simulink model "Dynamixel_Control_Validation_SpeedMode_2023a"  (R2023a)
settings: Solver=ode4  StartTime=0.0  StopTime=10  FixedStep=0.01  RelTol=1e-6  AbsTol=1e-6
undefined symbols (not defined in the file or in its folder): DiscIntNeverNeededParam
libraries: simulink x3, nvidiaSharedBlocks x1
settings Model: PauseTimes=45  Creator=SPOT  LastModifiedBy=SPOT
settings OptimizationCC: EnhancedBackFolding=on  PassReuseOutputArgsAs=Individual arguments  ZeroExternalMemoryAtStartup=off  ZeroInternalMemoryAtStartup=off  MaxStackSize=64  OptimizeBlockOrder=speed  DifferentSizesBufferReuse=on  OptimizationCustomize=off  EfficientTunableParamExpr=on
settings DebuggingCC: ParameterTunabilityLossMsg=error
settings HardwareCC: ProdBitPerLong=64  ProdLargestAtomicInteger=LongLong  ProdLargestAtomicFloat=Double  ProdLongLongMode=on  ProdHWDeviceType=ARM Compatible->ARM 64-bit (LP64)
settings SFSimCC: MATLABDynamicMemAlloc=off
settings RTWCC: Description=Embedded Coder  SystemTargetFile=ert.tlc  HardwareBoard=NVIDIA Jetson  TLCOptions="-aInlineSetEventsForThisBaseRateFcn=TLC_FALSE -aSuppressMultiTaskScheduler=TLC_FALSE  -aRateBasedStepFcn=0"  TemplateMakefile=ert_default_tmf  TargetLang=C++
settings CodeAppCC: ForceParamTrailComments=on  IgnoreCustomStorageClasses=off  OperatorAnnotations=on  SimulinkDataObjDesc=on  SFDataObjDesc=on  InsertBlockDesc=on
settings ERTTargetCC: MatFileLogging=on  SupportContinuousTime=on  SupportVariableSizeSignals=on

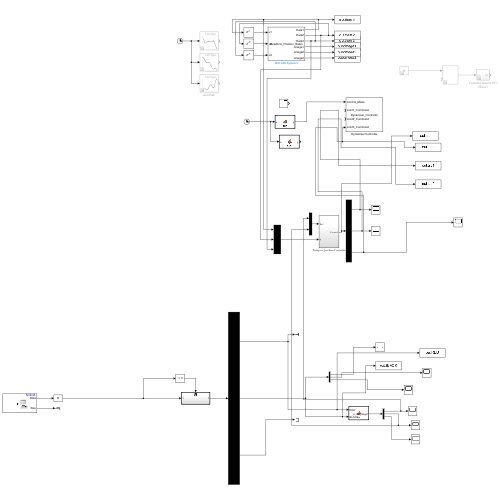
[thumbnail: Simulink's stored preview of the top-level diagram]
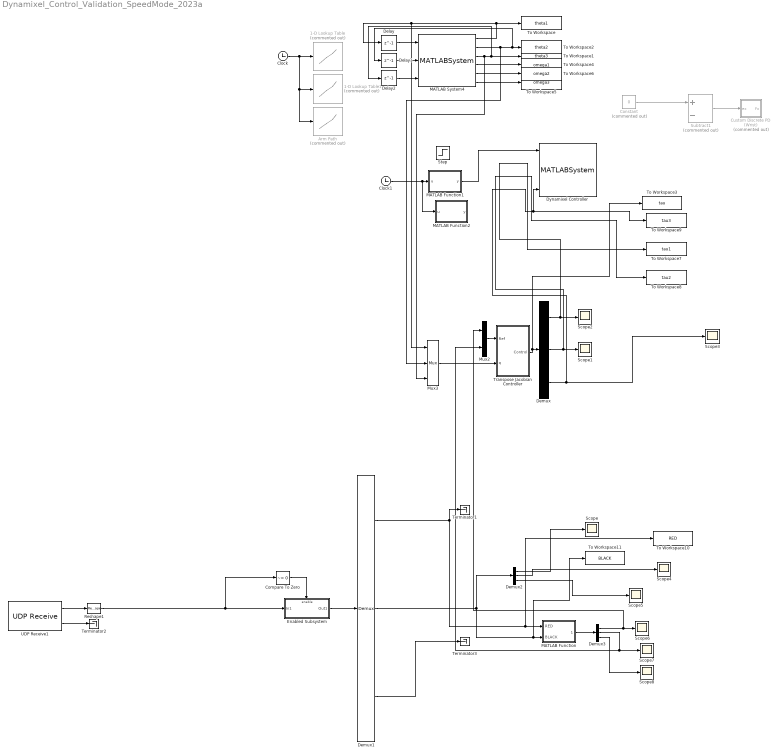
== system Dynamixel_Control_Validation_SpeedMode_2023a ==
  1-D Lookup Table : Lookup_n-D  Commented=on  NumberOfTableDimensions=1  BreakpointsForDimension1=|  Table=|  InternalRulePriority=Speed  RndMeth=Simplest
      BreakpointsForDimension1=|
      | [0
      | 0.300000000000000
      | 0.600000000000000
      | 0.900000000000000
      | 1.20000000000000
      | 1.50000000000000
      | 1.80000000000000
      | 2.10000000000000
      | 2.40000000000000
      | 2.70000000000000
      | 3
      | 3.30000000000000
      | 3.60000000000000
      | 3.90000000000000
      | 4.20000000000000
      | 4.50000000000000
      | 4.80000000000000
      | 5.10000000000000
      | 5.40000000000000
      | 5.70000000000000
      | 6
      | 6.30000000000000
      | 6.60000000000000
      | 6.90000000000000
      | 7.20000000000000
      | 7.50000000000000
      | 7.80000000000000
      | 8.10000000000000
      | 8.40000000000000
      | 8.70000000000000
      | 9
      | 9.30000000000000
      | 9.60000000000000
      | 9.90000000000000
      | 10.2000000000000
      | 10.5000000000000
      | 10.8000000000000
      | 11.1000000000000
      | 11.4000000000000
      | 11.7000000000000
      | 12
      | 12.3000000000000
      | 12.6000000000000
      | 12.9000000000000
      | 13.2000000000000
      | 13.5000000000000
      | 13.8000000000000
      | 14.1000000000000
      | 14.4000000000000
      | 14.7000000000000
      | 15
      | 15.3000000000000
      | 15.6000000000000
      | 15.9000000000000
      | 16.2000000000000
      | 16.5000000000000
      | 16.8000000000000
      | 17.1000000000000
      | 17.4000000000000
      | 17.7000000000000
      | 18
      | 18.3000000000000
      | 18.6000000000000
      | 18.9000000000000
      | 19.2000000000000
      | 19.5000000000000
      | 19.8000000000000
      | 20.1000000000000
      | 20.4000000000000
      | 20.7000000000000
      | 21
      | 21.3000000000000
      | 21.6000000000000
      | 21.9000000000000
      | 22.2000000000000
      | 22.5000000000000
      | 22.8000000000000
      | 23.1000000000000
      | 23.4000000000000
      | 23.7000000000000
      | 24
      | 24.3000000000000
      | 24.6000000000000
      | 24.9000000000000
      | 25.2000000000000
      | 25.5000000000000
      | 25.8000000000000
      | 26.1000000000000
      | 26.4000000000000
      | 26.7000000000000
      | 27
      | 27.3000000000000
      | 27.6000000000000
      | 27.9000000000000
      | 28.2000000000000
      | 28.5000000000000
      | 28.8000000000000
      | 29.1000000000000
      | 29.4000000000000
      | 29.7000000000000
      | 30]
      Table=|
      | [1.57000000000000
      | 1.54816700100684
      | 1.49097838714515
      | 1.40738374526561
      | 1.30517963261499
      | 1.19037595061406
      | 1.06817443571262
      | 0.943755752477061
      | 0.821348547944454
      | 0.703746844506339
      | 0.593625926874354
      | 0.493661079760138
      | 0.406301951764504
      | 0.332150464577563
      | 0.270904238844892
      | 0.222254718367453
      | 0.185893346946205
      | 0.161510391400890
      | 0.148507079640713
      | 0.145619174532266
      | 0.151489118608687
      | 0.164759354403110
      | 0.184072324448674
      | 0.208070471278512
      | 0.235433340233479
      | 0.265163793185692
      | 0.296431328827974
      | 0.328406827894775
      | 0.360261171120541
      | 0.391165239239719
      | 0.420289912986756
      | 0.446835197706220
      | 0.470407808441224
      | 0.490913309071205
      | 0.508264171683338
      | 0.522372868364801
      | 0.533151871202771
      | 0.540513652284423
      | 0.544370683696935
      | 0.544708678506983
      | 0.541826697403650
      | 0.536107583537685
      | 0.527934180942696
      | 0.517689333652287
      | 0.505755885700064
      | 0.492516681119634
      | 0.478354564411779
      | 0.463677280032886
      | 0.448984347405091
      | 0.434796424940426
      | 0.421634171050923
      | 0.410018244148617
      | 0.400469302645538
      | 0.393508004953720
      | 0.389655009485195
      | 0.389318793355856
      | 0.392420798366228
      | 0.398750326166947
      | 0.408096675929411
      | 0.420249146825022
      | 0.434997038025178
      | 0.452129648701280
      | 0.471436276672662
      | 0.492577909508950
      | 0.514735652583953
      | 0.536978444975800
      | 0.558375225762617
      | 0.577994934022531
      | 0.594906508833669
      | 0.608178889274159
      | 0.616885200503004
      | 0.620279657398225
      | 0.617862923664403
      | 0.609153311284521
      | 0.593669132241562
      | 0.570928698518508
      | 0.540450322098342
      | 0.501754708369804
      | 0.454651142688837
      | 0.399508826722755
      | 0.336761216407457
      | 0.266841767678842
      | 0.190183936472810
      | 0.107221178725261
      | 0.0184637402812976
      | -0.0750305460272099
      | -0.171966007758580
      | -0.271046003976081
      | -0.370973893742981
      | -0.470452548764951
      | -0.568113490727538
      | -0.662442454298735
      | -0.751907371290790
      | -0.834976173515947
      | -0.910130221885170
      | -0.976013131751286
      | -1.03137619058426
      | -1.07497442671845
      | -1.10593044052833
      | -1.12417944460303
      | -1.13000000000000]
  1-D Lookup Table1 : Lookup_n-D  Commented=on  NumberOfTableDimensions=1  BreakpointsForDimension1=|  Table=|  InternalRulePriority=Speed  RndMeth=Simplest
      BreakpointsForDimension1=|
      | [0
      | 0.300000000000000
      | 0.600000000000000
      | 0.900000000000000
      | 1.20000000000000
      | 1.50000000000000
      | 1.80000000000000
      | 2.10000000000000
      | 2.40000000000000
      | 2.70000000000000
      | 3
      | 3.30000000000000
      | 3.60000000000000
      | 3.90000000000000
      | 4.20000000000000
      | 4.50000000000000
      | 4.80000000000000
      | 5.10000000000000
      | 5.40000000000000
      | 5.70000000000000
      | 6
      | 6.30000000000000
      | 6.60000000000000
      | 6.90000000000000
      | 7.20000000000000
      | 7.50000000000000
      | 7.80000000000000
      | 8.10000000000000
      | 8.40000000000000
      | 8.70000000000000
      | 9
      | 9.30000000000000
      | 9.60000000000000
      | 9.90000000000000
      | 10.2000000000000
      | 10.5000000000000
      | 10.8000000000000
      | 11.1000000000000
      | 11.4000000000000
      | 11.7000000000000
      | 12
      | 12.3000000000000
      | 12.6000000000000
      | 12.9000000000000
      | 13.2000000000000
      | 13.5000000000000
      | 13.8000000000000
      | 14.1000000000000
      | 14.4000000000000
      | 14.7000000000000
      | 15
      | 15.3000000000000
      | 15.6000000000000
      | 15.9000000000000
      | 16.2000000000000
      | 16.5000000000000
      | 16.8000000000000
      | 17.1000000000000
      | 17.4000000000000
      | 17.7000000000000
      | 18
      | 18.3000000000000
      | 18.6000000000000
      | 18.9000000000000
      | 19.2000000000000
      | 19.5000000000000
      | 19.8000000000000
      | 20.1000000000000
      | 20.4000000000000
      | 20.7000000000000
      | 21
      | 21.3000000000000
      | 21.6000000000000
      | 21.9000000000000
      | 22.2000000000000
      | 22.5000000000000
      | 22.8000000000000
      | 23.1000000000000
      | 23.4000000000000
      | 23.7000000000000
      | 24
      | 24.3000000000000
      | 24.6000000000000
      | 24.9000000000000
      | 25.2000000000000
      | 25.5000000000000
      | 25.8000000000000
      | 26.1000000000000
      | 26.4000000000000
      | 26.7000000000000
      | 27
      | 27.3000000000000
      | 27.6000000000000
      | 27.9000000000000
      | 28.2000000000000
      | 28.5000000000000
      | 28.8000000000000
      | 29.1000000000000
      | 29.4000000000000
      | 29.7000000000000
      | 30]
      Table=|
      | [1.57000000000000
      | 1.57050205302399
      | 1.57012603662556
      | 1.56661162770156
      | 1.55794488562962
      | 1.54285929753597
      | 1.52042643744410
      | 1.48973080887809
      | 1.45048425411524
      | 1.40334397159352
      | 1.34904540279350
      | 1.28832398919572
      | 1.22195859634965
      | 1.15108368811919
      | 1.07700776270488
      | 1.00104050705195
      | 0.924491608105622
      | 0.848670299127955
      | 0.774774399465782
      | 0.703745216061739
      | 0.636488084287358
      | 0.573908339514172
      | 0.516911317113714
      | 0.466402352457517
      | 0.423202448662068
      | 0.387397731516399
      | 0.358695572215780
      | 0.336800200665272
      | 0.321415846769937
      | 0.312246740434836
      | 0.308997111565029
      | 0.311335869993361
      | 0.318438699519253
      | 0.329118863211428
      | 0.342181246399115
      | 0.356430734411547
      | 0.370672212577955
      | 0.383710566227569
      | 0.394350680689622
      | 0.401518359647600
      | 0.404656733001405
      | 0.403347252632020
      | 0.397171371877986
      | 0.385710544077849
      | 0.368546222570152
      | 0.345259860693440
      | 0.315432914518483
      | 0.278792464474893
      | 0.235602325706072
      | 0.186249942164213
      | 0.131122757801505
      | 0.0706082165701402
      | 0.00509376242231024
      | -0.0650331606897945
      | -0.139385108813982
      | -0.217505825480346
      | -0.298640304539486
      | -0.381952484472539
      | -0.466606302239867
      | -0.551765694801835
      | -0.636594599118806
      | -0.720256952151143
      | -0.801916690711806
      | -0.880723763116082
      | -0.955775800494991
      | -1.02615820551012
      | -1.09095638082305
      | -1.14925572909537
      | -1.20014165298867
      | -1.24269955516454
      | -1.27602769714638
      | -1.29978061439030
      | -1.31436988730625
      | -1.32026130853269
      | -1.31792067070809
      | -1.30781376647092
      | -1.29040638845964
      | -1.26616853457129
      | -1.23607724309064
      | -1.20209333571039
      | -1.16629053007224
      | -1.13074254381788
      | -1.09752309458901
      | -1.06870590002731
      | -1.04630359496360
      | -1.03189323418052
      | -1.02686268208325
      | -1.03259903268412
      | -1.05048937999544
      | -1.08191093831646
      | -1.12679451437392
      | -1.18211552054693
      | -1.24448846973170
      | -1.31052787482445
      | -1.37689087303085
      | -1.44074960138572
      | -1.49961795103105
      | -1.55095978791926
      | -1.58081445088490
      | -1.54996443310863
      | -1.48000000000000]
  Arm Path : Lookup_n-D  Commented=on  NumberOfTableDimensions=1  BreakpointsForDimension1=|  Table=|  InternalRulePriority=Speed  RndMeth=Simplest
      BreakpointsForDimension1=|
      | [0
      | 0.300000000000000
      | 0.600000000000000
      | 0.900000000000000
      | 1.20000000000000
      | 1.50000000000000
      | 1.80000000000000
      | 2.10000000000000
      | 2.40000000000000
      | 2.70000000000000
      | 3
      | 3.30000000000000
      | 3.60000000000000
      | 3.90000000000000
      | 4.20000000000000
      | 4.50000000000000
      | 4.80000000000000
      | 5.10000000000000
      | 5.40000000000000
      | 5.70000000000000
      | 6
      | 6.30000000000000
      | 6.60000000000000
      | 6.90000000000000
      | 7.20000000000000
      | 7.50000000000000
      | 7.80000000000000
      | 8.10000000000000
      | 8.40000000000000
      | 8.70000000000000
      | 9
      | 9.30000000000000
      | 9.60000000000000
      | 9.90000000000000
      | 10.2000000000000
      | 10.5000000000000
      | 10.8000000000000
      | 11.1000000000000
      | 11.4000000000000
      | 11.7000000000000
      | 12
      | 12.3000000000000
      | 12.6000000000000
      | 12.9000000000000
      | 13.2000000000000
      | 13.5000000000000
      | 13.8000000000000
      | 14.1000000000000
      | 14.4000000000000
      | 14.7000000000000
      | 15
      | 15.3000000000000
      | 15.6000000000000
      | 15.9000000000000
      | 16.2000000000000
      | 16.5000000000000
      | 16.8000000000000
      | 17.1000000000000
      | 17.4000000000000
      | 17.7000000000000
      | 18
      | 18.3000000000000
      | 18.6000000000000
      | 18.9000000000000
      | 19.2000000000000
      | 19.5000000000000
      | 19.8000000000000
      | 20.1000000000000
      | 20.4000000000000
      | 20.7000000000000
      | 21
      | 21.3000000000000
      | 21.6000000000000
      | 21.9000000000000
      | 22.2000000000000
      | 22.5000000000000
      | 22.8000000000000
      | 23.1000000000000
      | 23.4000000000000
      | 23.7000000000000
      | 24
      | 24.3000000000000
      | 24.6000000000000
      | 24.9000000000000
      | 25.2000000000000
      | 25.5000000000000
      | 25.8000000000000
      | 26.1000000000000
      | 26.4000000000000
      | 26.7000000000000
      | 27
      | 27.3000000000000
      | 27.6000000000000
      | 27.9000000000000
      | 28.2000000000000
      | 28.5000000000000
      | 28.8000000000000
      | 29.1000000000000
      | 29.4000000000000
      | 29.7000000000000
      | 30]
      Table=|
      | [4.24105195407198e-14
      | 0.00792484586540242
      | 0.0289766808051712
      | 0.0591226460349239
      | 0.0945266677508536
      | 0.132723049258546
      | 0.171865961865416
      | 0.210118613330810
      | 0.245977670299252
      | 0.278442298917847
      | 0.306553255045181
      | 0.329351294539841
      | 0.345978769405532
      | 0.356409999236062
      | 0.361026479142565
      | 0.360212485455902
      | 0.354352294506931
      | 0.343830913350855
      | 0.329212797758318
      | 0.311475554957133
      | 0.291654729751521
      | 0.270785866945703
      | 0.249904511343898
      | 0.230046207750326
      | 0.212190891231227
      | 0.196833909602021
      | 0.184220855187696
      | 0.174595248907400
      | 0.168200611680283
      | 0.165280464425496
      | 0.166078328062186
      | 0.170819192753770
      | 0.179469276510222
      | 0.191804652485855
      | 0.207596998435017
      | 0.226617992112058
      | 0.248639311271326
      | 0.273432633667171
      | 0.300769637053943
      | 0.330372138422153
      | 0.361748634952746
      | 0.394350586665731
      | 0.427629452980086
      | 0.461036693314793
      | 0.494023767088832
      | 0.526042133721183
      | 0.556543253290674
      | 0.585013755003088
      | 0.611069892609436
      | 0.634357776934821
      | 0.654523518804344
      | 0.671213229043108
      | 0.684073018476216
      | 0.692748997928769
      | 0.696887278225870
      | 0.696239394653257
      | 0.691014582997561
      | 0.681546260210274
      | 0.668167845572800
      | 0.651212758366539
      | 0.631014417872893
      | 0.607906243373263
      | 0.582221655279522
      | 0.554401355144190
      | 0.525287277542556
      | 0.495815140112214
      | 0.466920660490759
      | 0.439539556315785
      | 0.414607545224887
      | 0.393060344855659
      | 0.375828988968287
      | 0.363641886942561
      | 0.356951692355833
      | 0.356191311825241
      | 0.361793651967925
      | 0.374191619401025
      | 0.393818120741680
      | 0.421102648855173
      | 0.456063090510969
      | 0.497918715134657
      | 0.545797145289127
      | 0.598826003537267
      | 0.656132912441967
      | 0.716845494566115
      | 0.780034633378752
      | 0.844366607241886
      | 0.908331957834384
      | 0.970420511226358
      | 1.02912209348792
      | 1.08292634428082
      | 1.13029561275212
      | 1.16963648628818
      | 1.19934874289962
      | 1.21783216059706
      | 1.22367347867057
      | 1.21771835926845
      | 1.20231148671538
      | 1.17980152164021
      | 1.14786929261614
      | 1.09387618894762
      | 1.04000000000000]
  Clock : Clock
  Clock1 : Clock
  Compare To Zero : simulink/Logic and Bit Operations/Compare To Zero  relop=~=  OutDataTypeStr=boolean
  Constant : Constant  Commented=on  Value=0
  Custom Discrete PD (Wrist) : Subsystem  Commented=on
  Delay : Delay  DelayLength=1
  Delay1 : Delay  DelayLength=1
  Delay2 : Delay  DelayLength=1
  Demux : Demux  Outputs=3
  Demux1 : Demux  Outputs=[4,3,3]
  Demux2 : Demux  Outputs=3
  Demux3 : Demux  Outputs=3
  Dynamixel Controller : MATLABSystem  System=Dynamixel_Controller  POSITION_P_GAIN=400  POSITION_I_GAIN=0  POSITION_D_GAIN=200  MAX_POSITION=3072  MIN_POSITION=1024  MOVE_TIME=0  CURRENT_LIMIT=850  SPEED_P_GAIN=400  SPEED_I_GAIN=100  VELOCITY_LIMIT=50  ACCELERATION_TIME=0  SampleTime=0.01
      mask Type: Dynamixel_Controller
      mask Display:
      | disp('Dynamixel_Controller');
      | port_label('input',1,'Control_Mode');
      | port_label('input',2,'Joint1_Command');
      | port_label('input',3,'Joint2_Command');
      | port_label('input',4,'Joint3_Command');
  Enabled Subsystem : Subsystem  TreatAsAtomicUnit=on
  MATLAB Function : MATLAB Function  TreatAsAtomicUnit=on
  MATLAB Function1 : MATLAB Function  TreatAsAtomicUnit=on
  MATLAB Function2 : MATLAB Function  TreatAsAtomicUnit=on
  MATLAB System4 : MATLABSystem  System=ReadArm_Position_Rates  SampleTime=0.01
      mask Type: ReadArm_Position_Rates
      mask Display:
      | disp('ReadArm_Position_Rates');
      | port_label('input',1,'u1');
      | port_label('input',2,'u2');
      | port_label('input',3,'u3');
      | port_label('output',1,'theta1');
      | port_label('output',2,'theta2');
      | port_label('output',3,'theta3');
      | port_label('output',4,'omega1');
      | port_label('output',5,'omega2');
      | port_label('output',6,'omega3');
  Mux2 : Mux  Inputs=2
  Mux3 : Mux  Inputs=3
  Reshape1 : Reshape  OutputDimensionality=Customize  OutputDimensions=[10,1]
  Scope{,1..8} (9 alike) : Scope
  Step : Step  Time=0.3  After=3  SampleTime=0
  Subtract1 : Sum  Commented=on  Inputs=+-
  Terminator1 : Terminator
  Terminator2 : Terminator
  Terminator3 : Terminator
  To Workspace : ToWorkspace  VariableName=theta1  SampleTime=-1
      settings: Save2DSignal=2-D array (concatenate along first dimension)
  To Workspace1 : ToWorkspace  VariableName=theta3  SampleTime=-1
      settings: Save2DSignal=2-D array (concatenate along first dimension)
  To Workspace10 : ToWorkspace  VariableName=RED  SampleTime=-1
      settings: Save2DSignal=2-D array (concatenate along first dimension)
  To Workspace11 : ToWorkspace  VariableName=BLACK  SampleTime=-1
      settings: Save2DSignal=2-D array (concatenate along first dimension)
  To Workspace2 : ToWorkspace  VariableName=theta2  SampleTime=-1
      settings: Save2DSignal=2-D array (concatenate along first dimension)
  To Workspace3 : ToWorkspace  VariableName=tau  SampleTime=-1
      settings: Save2DSignal=2-D array (concatenate along first dimension)
  To Workspace4 : ToWorkspace  VariableName=omega1  SampleTime=-1
      settings: Save2DSignal=2-D array (concatenate along first dimension)
  To Workspace5 : ToWorkspace  VariableName=omega3  SampleTime=-1
      settings: Save2DSignal=2-D array (concatenate along first dimension)
  To Workspace6 : ToWorkspace  VariableName=omega2  SampleTime=-1
      settings: Save2DSignal=2-D array (concatenate along first dimension)
  To Workspace7 : ToWorkspace  VariableName=tau1  SampleTime=-1
      settings: Save2DSignal=2-D array (concatenate along first dimension)
  To Workspace8 : ToWorkspace  VariableName=tau2  SampleTime=-1
      settings: Save2DSignal=2-D array (concatenate along first dimension)
  To Workspace9 : ToWorkspace  VariableName=tau3  SampleTime=-1
      settings: Save2DSignal=2-D array (concatenate along first dimension)
  Transpose Jacobian Controller : Subsystem
  UDP Receive1 : nvidiaSharedBlocks/UDP Receive  localURL='0.0.0.0'  localPort=31534  remoteURL='0.0.0.0'  remotePort=-1  recvBufferSize=8192  signalDatatype=double  dims=10  isVarSize=off  showBlockingTime=off  blockingTime=0  sampletime=-1  blockPlatform=NVIDIA
  wires:
  Demux/1 -> To Workspace7/1, Scope2/1
  MATLAB System4/4 -> To Workspace4/1
  Mux3/1 -> Transpose Jacobian Controller/2(q)
  Mux2/1 -> Transpose Jacobian Controller/1(Ref)
  Demux3/2 -> Scope7/1, Mux2/2
  Clock/1 -> Arm Path/1, 1-D Lookup Table1/1, 1-D Lookup Table/1
  Demux3/1 -> Mux2/1, Scope6/1
  MATLAB System4/6 -> To Workspace5/1
  Compare To Zero/1 -> Enabled Subsystem/Enable
  MATLAB System4/2 -> Mux3/2, Delay1/1, To Workspace2/1
  Demux1/2 -> Demux2/1, To Workspace11/1, MATLAB Function/2(BLACK)
  Demux2/3 -> Scope5/1
  Demux2/1 -> Scope/1
  Delay1/1 -> MATLAB System4/2
  Delay/1 -> MATLAB System4/1
  Demux2/2 -> Scope4/1
  Demux1/3 -> Terminator3/1
  Demux3/3 -> Scope8/1
  MATLAB System4/3 -> Mux3/3, Delay2/1, To Workspace1/1
  MATLAB Function/1(p_red_target) -> Demux3/1
  Constant/1 -> Subtract1/1
  MATLAB System4/1 -> Mux3/1, Delay/1, To Workspace/1
  Subtract1/1 -> Custom Discrete PD (Wrist)/1(ex)
  Demux/2 -> To Workspace8/1, Scope1/1
  Enabled Subsystem/1(Out1) -> Demux1/1
  Delay2/1 -> MATLAB System4/3
  MATLAB System4/5 -> To Workspace6/1
  Reshape1/1 -> Enabled Subsystem/1(In1), Compare To Zero/1
  UDP Receive1/1 -> Reshape1/1
  Demux1/1 -> Terminator1/1, To Workspace10/1, MATLAB Function/1(RED)
  UDP Receive1/2 -> Terminator2/1
  Demux/3 -> Dynamixel Controller/4, To Workspace9/1, Scope3/1
  Transpose Jacobian Controller/1(Control) -> To Workspace3/1, Demux/1
  Clock1/1 -> MATLAB Function2/1(u), MATLAB Function1/1(u)
  MATLAB Function1/1(y) -> Dynamixel Controller/1

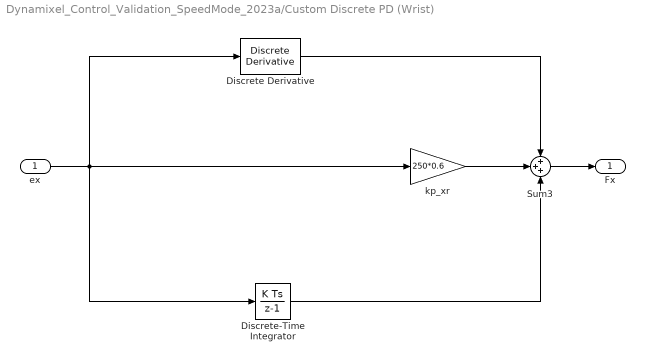
== system Dynamixel_Control_Validation_SpeedMode_2023a/Custom Discrete PD (Wrist) ==
  ex : Inport
  Discrete Derivative : simulink/Discrete/Discrete Derivative  gainval=0  ICPrevScaledInput=0.0  OutMin=[]  OutMax=[]  OutDataType=fixdt(1, 16)  OutScaling=2^-10  DoSatur=off
  Discrete-Time Integrator : DiscreteIntegrator  gainval=100  SampleTime=-1  ICPrevOutput=DiscIntNeverNeededParam  ICPrevScaledInput=DiscIntNeverNeededParam
  Sum3 : Sum  Inputs=+++
  kp_xr : Gain  Gain=250*0.6
  Fx : Outport  VectorParamsAs1DForOutWhenUnconnected=off
  wires:
  Discrete Derivative/1 -> Sum3/1
  ex/1 -> Discrete-Time Integrator/1, kp_xr/1, Discrete Derivative/1
  kp_xr/1 -> Sum3/2
  Sum3/1 -> Fx/1
  Discrete-Time Integrator/1 -> Sum3/3

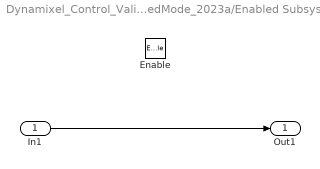
== system Dynamixel_Control_Validation_SpeedMode_2023a/Enabled Subsystem ==
  In1 : Inport
  Enable : EnablePort
  Out1 : Outport  VectorParamsAs1DForOutWhenUnconnected=off
  wires:
  In1/1 -> Out1/1

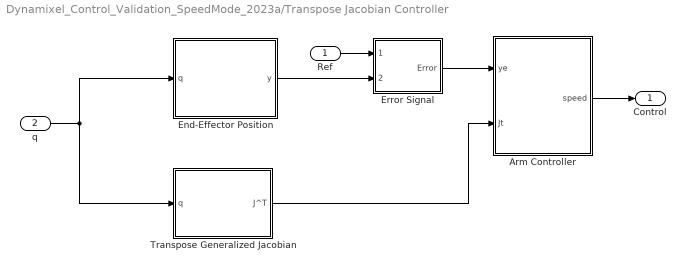
== system Dynamixel_Control_Validation_SpeedMode_2023a/Transpose Jacobian Controller ==
  Ref : Inport
  q : Inport  Port=2
  Arm Controller : Subsystem
  End-Effector Position : MATLAB Function  TreatAsAtomicUnit=on
  Error Signal : Subsystem
  "Transpose Generalized Jacobian " : Subsystem
  Control : Outport  VectorParamsAs1DForOutWhenUnconnected=off
  wires:
  Ref/1 -> Error Signal/1(Reference)
  End-Effector Position/1(y) -> Error Signal/2(Current)
  q/1 -> End-Effector Position/1(q), "Transpose Generalized Jacobian "/1(q)
  "Transpose Generalized Jacobian "/1(J^T) -> Arm Controller/2(Jt)
  Error Signal/1(Error) -> Arm Controller/1(ye)
  Arm Controller/1(speed) -> Control/1

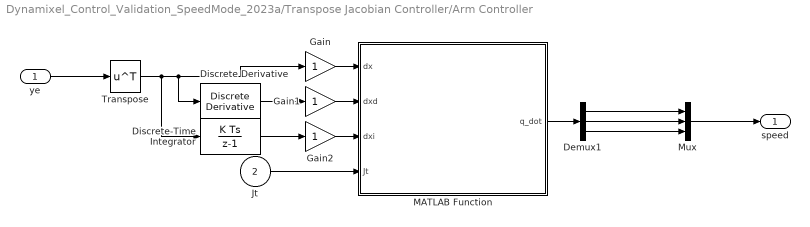
== system Dynamixel_Control_Validation_SpeedMode_2023a/Transpose Jacobian Controller/Arm Controller ==
  ye : Inport
  Jt : Inport  Port=2
  Demux1 : Demux  Outputs=3
  Discrete Derivative : simulink/Discrete/Discrete Derivative  gainval=1.0  ICPrevScaledInput=0.0  OutMin=[]  OutMax=[]  OutDataType=fixdt(1, 16)  OutScaling=2^-10  DoSatur=off
  Discrete-Time Integrator : DiscreteIntegrator  SampleTime=-1  ICPrevOutput=DiscIntNeverNeededParam  ICPrevScaledInput=DiscIntNeverNeededParam
  Gain : Gain
  Gain1 : Gain
  Gain2 : Gain
  MATLAB Function : MATLAB Function  TreatAsAtomicUnit=on
  Mux : Mux  Inputs=3
  Transpose : Math  Operator=transpose
  speed : Outport  VectorParamsAs1DForOutWhenUnconnected=off
  wires:
  ye/1 -> Transpose/1
  Jt/1 -> MATLAB Function/4(Jt)
  Discrete Derivative/1 -> Gain1/1
  Discrete-Time Integrator/1 -> Gain2/1
  MATLAB Function/1(q_dot) -> Demux1/1
  Demux1/1 -> Mux/1
  Demux1/2 -> Mux/2
  Demux1/3 -> Mux/3
  Mux/1 -> speed/1
  Gain/1 -> MATLAB Function/1(dx)
  Gain1/1 -> MATLAB Function/2(dxd)
  Gain2/1 -> MATLAB Function/3(dxi)
  Transpose/1 -> Discrete-Time Integrator/1, Discrete Derivative/1, Gain/1

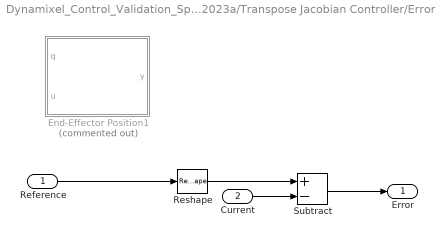
== system Dynamixel_Control_Validation_SpeedMode_2023a/Transpose Jacobian Controller/Error Signal ==
  Reference : Inport
  Current : Inport  Port=2
  End-Effector Position1 : MATLAB Function  Commented=on  TreatAsAtomicUnit=on
  Reshape : Reshape  OutputDimensionality=Row vector (2-D)
  Subtract : Sum  Inputs=+-
  Error : Outport  VectorParamsAs1DForOutWhenUnconnected=off
  wires:
  Subtract/1 -> Error/1
  Current/1 -> Subtract/2
  Reshape/1 -> Subtract/1
  Reference/1 -> Reshape/1

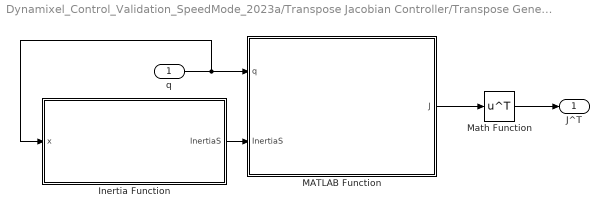
== system Dynamixel_Control_Validation_SpeedMode_2023a/Transpose Jacobian Controller/Transpose Generalized Jacobian  ==
  q : Inport
  "Inertia Function " : MATLAB Function  TreatAsAtomicUnit=on
  MATLAB Function : MATLAB Function  TreatAsAtomicUnit=on
  Math Function : Math  Operator=transpose  SignedPower=on
  J^T : Outport  VectorParamsAs1DForOutWhenUnconnected=off
  wires:
  Math Function/1 -> J^T/1
  q/1 -> "Inertia Function "/1(x), MATLAB Function/1(q)
  MATLAB Function/1(J) -> Math Function/1
  "Inertia Function "/1(InertiaS) -> MATLAB Function/2(InertiaS)

== matlab function Dynamixel_Control_Validation_SpeedMode_2023a/MATLAB Function1 ==
  data: u input; y output
function y = fcn(u)

    if u < 2
        y = 0;
    elseif u >= 2 && u < 5
        y = 3;
    elseif u >= 5 && u < 7
        y = 0;
    elseif u >= 7
        y = 1;
    else 
        y = 0;
    end


end

== matlab function Dynamixel_Control_Validation_SpeedMode_2023a/MATLAB Function ==
  data: RED input; p_red_target output; BLACK input
function p_red_target = fcn(RED, BLACK)

    Pi_red_x = RED(2)/1000;
    Pi_red_y = RED(3)/1000;
    Pi_red_theta = RED(4);
    Pi_black_x = BLACK(1)/1000;
    Pi_black_y = BLACK(2)/1000;
    Pi_black_theta = BLACK(3); 
    
    % Define the rotation matrices for the first and second satellites
    R_red = [cos(Pi_red_theta) -sin(Pi_red_theta) 0; sin(Pi_red_theta) cos(Pi_red_theta) 0; 0 0 1];
    R_black = [cos(Pi_black_theta) -sin(Pi_black_theta) 0; sin(Pi_black_theta) cos(Pi_black_theta) 0; 0 0 1];

    % Define the offset vector for the target location
    v_target_body = [0.0743; 0.2288; 0];

    % Rotate the offset vector into the inertial frame
    v_target_inertial = R_black * v_target_body;

    % Compute the position of the center of mass of the second satellite in the inertial frame
    p_black_inertial = [Pi_black_x; Pi_black_y; 0] + v_target_inertial;

    % Compute the position of the center of mass of the second satellite in the first satellite's frame
    p_black_relative = R_red' * (p_black_inertial - [Pi_red_x; Pi_red_y; 0]);

    % Compute the position of the target in the first satellite's frame
    p_red_target = p_black_relative;


end

== matlab function Dynamixel_Control_Validation_SpeedMode_2023a/MATLAB Function2 ==
  data: u input; y output
function y = fcn(u)

    if u < 2
        y = 0;
    elseif u >= 2 && u < 5
        y = -20;
    elseif u >= 5 && u < 7
        y = 0;
    elseif u >= 7
        y = 0;
    else
        y = 0;
    end


end

== matlab function Dynamixel_Control_Validation_SpeedMode_2023a/Transpose Jacobian Controller/Arm Controller/MATLAB Function ==
  data: dx input; dxd input; dxi input; q_dot output; Jt input
function q_dot  = fcn(dx, dxd, dxi, Jt)
    %#codegen
    

    q_dot = Jt*(dx + dxi);
                   
end

== matlab function Dynamixel_Control_Validation_SpeedMode_2023a/Transpose Jacobian Controller/Error Signal/End-Effector Position1 ==
  data: y output; q input; u input
function y = ForwardKinematics(q, u)
%#codegen
theta = q(3);

C_bI_RED = [  cos(theta) sin(theta)
            -sin(theta) cos(theta) ];
                                 
y  = C_bI_RED*u;  
end

== matlab function Dynamixel_Control_Validation_SpeedMode_2023a/Transpose Jacobian Controller/End-Effector Position ==
  data: y output; q input
function y = ForwardKinematics(q)
%#codegen

phi= 73.2749*pi/180;          % ARM Phi
b0= 0.25;                     % ARM b0
a1= 0.196822;                 % ARM a1
b1= 0.107678;                 % ARM b1
a2= 0.198152;                 % ARM a2
b2= 0.106348;                 % ARM b2
a3= 0.062097;                 % ARM a3
b3= 0.025153;                 % ARM b3

l1     = a1+b1;
l2     = a2+b2;
l3     = a3+b3;

% Define Variables
q1 = q(1);
q2 = q(2);
q3 = q(3);

% Calculate End-Effector Position & Velocity
y = [ (b0)*cos(phi) + (l1)*cos(pi/2+q1) + (l2)*cos(pi/2+q1+q2) + (l3)*cos(pi/2+q1+q2+q3),...
      (b0)*sin(phi) + (l1)*sin(pi/2+q1) + (l2)*sin(pi/2+q1+q2) + (l3)*sin(pi/2+q1+q2+q3)];
  
end

== matlab function Dynamixel_Control_Validation_SpeedMode_2023a/Transpose Jacobian Controller/Transpose Generalized Jacobian /MATLAB Function ==
  data: q input; J output; InertiaS input
function J  = fcn(q, InertiaS)
%#codegen

% Source: http://ieeexplore.ieee.org.proxy.library.carleton.ca/stamp/stamp.jsp?tp=&arnumber=34766
q0 = 0;
q1     = q(1);
q2     = q(2);
q3     = q(3);

m0            = 13.0720;     % RED Mass
I0            = 0.2405;      % RED Inertia
phi           = 73.2749*180/pi; % ARM Phi
b0            = 0.25;        % ARM b0
a1            = 0.196822;    % ARM a1
b1            = 0.107678;    % ARM b1
a2            = 0.198152;    % ARM a2
b2            = 0.106348;    % ARM b2
a3            = 0.062097;    % ARM a3
b3            = 0.025153;    % ARM b3
m1            = 0.345;       % ARM m1
m2            = 0.335;       % ARM m2
m3            = 0.111;       % ARM m3
I1            = 0.003704;    % ARM I1
I2            = 0.003506;    % ARM I2
I3            = 0.000106;    % ARM I3
l1     = a1+b1;
l2     = a2+b2;
l3     = a3+b3;

w = m0+m1+m2+m3;

% J = [ 1, 0, - l3*sin(q0 + q1 + q2 + q3) - b0*sin(phi + q0) - l1*sin(q0 + q1) - l2*sin(q0 + q1 + q2), - l3*sin(q0 + q1 + q2 + q3) - l1*sin(q0 + q1) - l2*sin(q0 + q1 + q2), - l3*sin(q0 + q1 + q2 + q3) - l2*sin(q0 + q1 + q2), -l3*sin(q0 + q1 + q2 + q3)
%       0, 1,   l3*cos(q0 + q1 + q2 + q3) + b0*cos(phi + q0) + l1*cos(q0 + q1) + l2*cos(q0 + q1 + q2),   l3*cos(q0 + q1 + q2 + q3) + l1*cos(q0 + q1) + l2*cos(q0 + q1 + q2),   l3*cos(q0 + q1 + q2 + q3) + l2*cos(q0 + q1 + q2),  l3*cos(q0 + q1 + q2 + q3)];

% Contants
K0     = m0*b0/w;
K1     = (m0*l1 + m1*b1)/w;
K2     = ((m0+m1)*l2 + m2*b2)/w;
K3     = ((m0+m1+m2)*l3 + m3*b3)/w;

% Trigonometric simplifications
s0     = sin(phi);
s1     = sin(pi/2+q1);
s2     = sin(pi/2+q1+q2);
s3     = sin(pi/2+q1+q2+q3);
c0     = cos(phi);
c1     = cos(pi/2+q1);
c2     = cos(pi/2+q1+q2);
c3     = cos(pi/2+q1+q2+q3);

% Jacobian for the base (specific)       
Jm     = [ -K1*s1-K2*s2-K3*s3 -K2*s2-K3*s3 -K3*s3 
            K1*c1+K2*c2+K3*c3  K2*c2+K3*c3  K3*c3  ];

% Jacobian for the manipulator (specific)
Js     = [ -K0*b0*s0-K1*l1*s1-K2*l2*s2-K3*l3*s3
            K0*b0*c0+K1*l1*c1+K2*l2*c2+K3*l3*c3 ];

% More constants
H      = InertiaS;
                      
Is     = H(3,3);
Im     = [H(3,4), H(3,5), H(3,6)];

% Calculate generalized Jacobian
J      = Jm - Js*(Is\Im);  

end

== matlab function Dynamixel_Control_Validation_SpeedMode_2023a/Transpose Jacobian Controller/Transpose Generalized Jacobian /Inertia Function  ==
  data: InertiaS output; x input
function InertiaS = InertiaFunc3LINK(x)
%INERTIAFUNC3LINK
%    INERTIAS = INERTIAFUNC3LINK(I0,I1,I2,I3,A1,A2,A3,B0,B1,B2,M0,M1,M2,M3,PHI,Q0,Q1,Q2,Q3)

%    This function was generated by the Symbolic Math Toolbox version 8.5.
%    15-Mar-2022 15:58:51

q0 = 0;
q1 = x(1);
q2 = x(2);
q3 = x(3);

m0            = 13.0720;     % RED Mass
I0            = 0.2405;      % RED Inertia
phi           = 73.2749*180/pi; % ARM Phi
b0            = 0.25;        % ARM b0
a1            = 0.196822;    % ARM a1
b1            = 0.107678;    % ARM b1
a2            = 0.198152;    % ARM a2
b2            = 0.106348;    % ARM b2
a3            = 0.062097;    % ARM a3
b3            = 0.025153;    % ARM b3
m1            = 0.345;       % ARM m1
m2            = 0.335;       % ARM m2
m3            = 0.111;       % ARM m3
I1            = 0.003704;    % ARM I1
I2            = 0.003506;    % ARM I2
I3            = 0.000106;    % ARM I3

t2 = cos(q2);
t3 = cos(q3);
t4 = a1+b1;
t5 = a2+b2;
t6 = a1.*m1;
t7 = a2.*m2;
t8 = a2.*m3;
t9 = a3.*m3;
t10 = b0.*m1;
t11 = b0.*m2;
t12 = b0.*m3;
t13 = b2.*m3;
t14 = phi+q0;
t15 = q0+q1;
t16 = q2+q3;
t17 = a1.^2;
t18 = a2.^2;
t19 = a3.^2;
t20 = b0.^2;
t21 = b1.^2;
t22 = b2.^2;
t48 = -phi;
t49 = -q1;
t50 = m0+m1+m2+m3;
t76 = a1.*b1.*m2.*2.0;
t77 = a1.*b1.*m3.*2.0;
t23 = a1.*t7;
t24 = a1.*t8;
t25 = a1.*t9;
t26 = a3.*t8;
t27 = b0.*t6;
t28 = a1.*t11;
t29 = a1.*t12;
t30 = b0.*t7;
t31 = b0.*t8;
t32 = b1.*t7;
t33 = a1.*t13;
t34 = b1.*t8;
t35 = b0.*t9;
t36 = b1.*t9;
t37 = b2.*t9;
t38 = b1.*t11;
t39 = b1.*t12;
t40 = b2.*t12;
t41 = b1.*t13;
t42 = cos(t14);
t43 = cos(t15);
t44 = cos(t16);
t45 = q2+t15;
t46 = sin(t14);
t47 = sin(t15);
t52 = t15+t16;
t54 = -t6;
t55 = -t7;
t56 = -t8;
t57 = -t9;
t58 = -t10;
t59 = -t11;
t60 = -t12;
t61 = -t13;
t62 = a1.*t6;
t63 = m2.*t17;
t64 = m3.*t17;
t65 = a2.*t7;
t66 = a2.*t8;
t67 = a3.*t9;
t69 = m2.*t21;
t70 = m3.*t21;
t71 = b2.*t13;
t81 = b2.*t8.*2.0;
t85 = m2.*t4;
t86 = m3.*t4;
t87 = m3.*t5;
t94 = phi+t49;
t95 = q1+q2+t48;
t101 = q1+t16+t48;
t106 = t10+t11+t12;
t51 = cos(t45);
t53 = sin(t45);
t68 = t67;
t72 = t23.*2.0;
t73 = t24.*2.0;
t74 = t25.*2.0;
t75 = t26.*2.0;
t78 = t32.*2.0;
t79 = t33.*2.0;
t80 = t34.*2.0;
t82 = t36.*2.0;
t83 = t37.*2.0;
t84 = t41.*2.0;
t88 = cos(t52);
t89 = -t30;
t90 = -t31;
t91 = -t35;
t92 = -t40;
t93 = sin(t52);
t96 = sin(t94);
t98 = -t85;
t99 = -t86;
t100 = -t87;
t102 = sin(t95);
t103 = t25+t36;
t104 = t26+t37;
t105 = sin(t101);
t115 = t42.*t106;
t118 = t55+t56+t61;
t119 = t58+t59+t60;
t125 = t27+t28+t29+t38+t39;
t126 = -t46.*t106;
t129 = -t43.*(t6+t85+t86);
t130 = -t47.*(t6+t85+t86);
t131 = t23+t24+t32+t33+t34+t41;
t97 = I3+t68;
t107 = t74+t82;
t108 = t75+t83;
t109 = t57.*t88;
t110 = t57.*t93;
t111 = t3.*t104;
t112 = t55+t100;
t113 = t44.*t103;
t117 = t91.*t105;
t120 = -t53.*(t7+t87);
t121 = t89+t90+t92;
t122 = -t51.*(t7+t87);
t124 = t54+t98+t99;
t127 = -t51.*(t7+t8+t13);
t128 = -t53.*(t7+t8+t13);
t133 = t2.*t131;
t134 = -t102.*(t30+t31+t40);
t135 = t96.*t125;
t136 = t72+t73+t78+t79+t80+t84;
t114 = t3.*t108;
t116 = t44.*t107;
t123 = t97+t111;
t132 = I2+t65+t66+t71+t81+t97;
t138 = t2.*t136;
t139 = t109+t127;
t140 = t110+t128;
t142 = t110+t120+t130;
t143 = t109+t122+t129;
t137 = t113+t123;
t144 = I1+t62+t63+t64+t69+t70+t76+t77+t132;
t145 = t115+t142;
t146 = t126+t143;
t147 = t113+t114+t132+t133;
t141 = t117+t137;
t148 = t117+t134+t147;
t149 = t114+t116+t117+t134+t135+t138+t144;
InertiaS = reshape([t50,0.0,t146,t143,t139,t109,0.0,t50,t145,t142,t140,t110,t146,t145,I0+t114+t116+t135.*2.0+t138+t144+b0.*t10+b0.*t11+b0.*t12-t35.*t105.*2.0-t102.*(t30.*2.0+t31.*2.0+t40.*2.0),t149,t148,t141,t143,t142,t149,t114+t116+t138+t144,t147,t137,t139,t140,t148,t147,t114+t132,t123,t109,t110,t141,t137,t123,t97],[6,6]);

end
